simulink model "Follower"  (R2024b)
settings: Solver=ode4  StartTime=0  StopTime=100  FixedStep=0.001  RelTol=1e-3
undefined symbols (not defined in the file or in its folder): DiscIntNeverNeededParam
libraries: simulink x22, vrlib x1
(part 4 of 4)

== matlab function Follower/Ardupilot Attitude Controller/Attitude Controller/input_euler_angle_roll_pitch_euler_rate_yaw()/Feedforward enabled/input shaping/input shaping pitch angle/Square Root Controller1/Square Root Controller ==
  data: err input; correction_rate output; p input; second_ord_lim input; dt input
function correction_rate = sqrt_controller(err, p, second_ord_lim, dt)
% The square root controller
% Code is taken from sqrt_controller(...) in AC_PosControl.cpp.

if (second_ord_lim < 0 || second_ord_lim == 0)
   correction_rate = err * p;
elseif (p == 0)
    % P term is zero, but second order limit is positive
    if (err > 0)
        correction_rate = sqrt(single(2.0) * second_ord_lim * err);
    elseif (err < 0)
        correction_rate = sqrt(single(2.0) * second_ord_lim * -err);
    else
        correction_rate = single(0.0);
    end
else
    % P term and second order limit are positive, hence have been defined
    linear_dist = second_ord_lim / (p * p);
    % Check if error exceeds linear range of controller gain
    if (err > linear_dist)
        correction_rate = sqrt(single(2.0) * second_ord_lim * ( err - (linear_dist / single(2.0)) ));
    elseif (err < -linear_dist)
        correction_rate = -sqrt(single(2.0) * second_ord_lim * ( -err - (linear_dist / single(2.0)) ));
    else
        % Return linearly amplified correction if error is in linear range
        correction_rate = err * p;
    end
end

% Prevent oscillations by over-shooting the error correction in the last
% time step
if (dt ~= 0)
    correction_rate = max( min(correction_rate, abs(err) / dt), -abs(err) / dt);
end

== matlab function Follower/Ardupilot Attitude Controller/Attitude Controller/input_euler_angle_roll_pitch_euler_rate_yaw()/Feedforward enabled/input shaping/input shaping roll angle/Square Root Controller1/Square Root Controller ==
  data: err input; correction_rate output; p input; second_ord_lim input; dt input
function correction_rate = sqrt_controller(err, p, second_ord_lim, dt)
% The square root controller
% Code is taken from sqrt_controller(...) in AC_PosControl.cpp.

if (second_ord_lim < 0 || second_ord_lim == 0)
   correction_rate = err * p;
elseif (p == 0)
    % P term is zero, but second order limit is positive
    if (err > 0)
        correction_rate = sqrt(single(2.0) * second_ord_lim * err);
    elseif (err < 0)
        correction_rate = sqrt(single(2.0) * second_ord_lim * -err);
    else
        correction_rate = single(0.0);
    end
else
    % P term and second order limit are positive, hence have been defined
    linear_dist = second_ord_lim / (p * p);
    % Check if error exceeds linear range of controller gain
    if (err > linear_dist)
        correction_rate = sqrt(single(2.0) * second_ord_lim * ( err - (linear_dist / single(2.0)) ));
    elseif (err < -linear_dist)
        correction_rate = -sqrt(single(2.0) * second_ord_lim * ( -err - (linear_dist / single(2.0)) ));
    else
        % Return linearly amplified correction if error is in linear range
        correction_rate = err * p;
    end
end

% Prevent oscillations by over-shooting the error correction in the last
% time step
if (dt ~= 0)
    correction_rate = max( min(correction_rate, abs(err) / dt), -abs(err) / dt);
end

== matlab function Follower/Ardupilot Attitude Controller/Attitude Controller/input_euler_angle_roll_pitch_euler_rate_yaw()/Feedforward enabled/input shaping/input shaping yaw rate/Square Root Controller/Square Root Controller ==
  data: err input; correction_rate output; p input; second_ord_lim input; dt input
function correction_rate = sqrt_controller(err, p, second_ord_lim, dt)
% The square root controller
% Code is taken from sqrt_controller(...) in AC_PosControl.cpp.

if (second_ord_lim < 0 || second_ord_lim == 0)
   correction_rate = err * p;
elseif (p == 0)
    % P term is zero, but second order limit is positive
    if (err > 0)
        correction_rate = sqrt(single(2.0) * second_ord_lim * err);
    elseif (err < 0)
        correction_rate = sqrt(single(2.0) * second_ord_lim * -err);
    else
        correction_rate = single(0.0);
    end
else
    % P term and second order limit are positive, hence have been defined
    linear_dist = second_ord_lim / (p * p);
    % Check if error exceeds linear range of controller gain
    if (err > linear_dist)
        correction_rate = sqrt(single(2.0) * second_ord_lim * ( err - (linear_dist / single(2.0)) ));
    elseif (err < -linear_dist)
        correction_rate = -sqrt(single(2.0) * second_ord_lim * ( -err - (linear_dist / single(2.0)) ));
    else
        % Return linearly amplified correction if error is in linear range
        correction_rate = err * p;
    end
end

% Prevent oscillations by over-shooting the error correction in the last
% time step
if (dt ~= 0)
    correction_rate = max( min(correction_rate, abs(err) / dt), -abs(err) / dt);
end

== matlab function Follower/Ardupilot Attitude Controller/MATLAB Function4 ==
  data: x input; phi_des output; xdes input; theta_des output; psidot_des output; Ux input; Uy input
function [phi_des, theta_des, psidot_des] = GetDesiredAttitude(x, xdes, Ux, Uy)
% Calculate phi and theta desired based on psi, Ux and Uy and limit them to
% +- pi/3
% xdes = [phi p theta q psi r x xdot y ydot z zdot]
angle_limit = 5*pi/12;

temp1 = Ux * sin(xdes(5)) - Uy * cos(xdes(5));
phi_des = asin(max(min(temp1, sin(angle_limit)), -sin(angle_limit)));

temp2 = (Ux - sin(xdes(1)) * sin(xdes(5))) / (cos(xdes(1)) * cos(xdes(5))); 
theta_des = asin(max(min(temp2, sin(angle_limit)), -sin(angle_limit)));

Kp_psi = 1.0;
psidot_des = Kp_psi * (xdes(5) - x(5));

== matlab function Follower/MATLAB Function5 ==
  data: V output; Z input
function V  = RotorModel(Z)

V = zeros(4,1);
V(1) = Z(1)^2/2;
V(2) = (V(1) + Z(2)^2)/2;
V(3) = Z(3)^2/2;
V(4) = (V(3) + Z(4)^2)/2;

== matlab function Follower/SMC Position Controller/MATLAB Function7 ==
  data: zintg input; x input; Sx output; Sy output; Sz output; Z output; xhat input; xdes input
function [Sx, Sy, Sz, Z] = SlidingSurfaces(zintg, x, xhat, xdes)

% xdes = (phi p theta q psi r x xdot y ydot z zdot)
alpha = 1.5;

z = zeros(12,1);
for i = 1:2:6
    z(i) = x(i) - xdes(i);
    
    % Using ground truth states
    % z(6 + i) = x(6 + i) - xdes(6 + i);
    % Using estimated states
    z(6 + i) = xhat(i) - xdes(6 + i);
end
for j = 2:2:6
    z(j) = x(j) - xdes(j) + alpha*z(j-1);
    
    % Using ground truth states
    % z(6 + j) = x(6 + j) - xdes(6 + j);
    % Using estimated states
    z(6 + j) = xhat(j) - xdes(6 + j);
end
Z = [z(1); z(2); z(3); z(4)];

% Normal SMC
Sx = z(8) + alpha*z(7);
Sy = z(10) + alpha*z(9);
% Sz = z(12) + alpha*z(11);

% Integral SMC
Sz = z(12) + 2*alpha*z(11) + alpha^2 * zintg;

== matlab function Follower/SMC Position Controller/MATLAB Function1 ==
  data: x input; xhat input; xdes input; xdesdot input; U1 output; Ux output; Uy output; Sx input; Sy input; Sz input; k1 output; kx output; ky output
function [U1, Ux, Uy, k1, kx, ky] = PositionController(x, xhat, xdes, xdesdot, Sx, Sy, Sz)

%initializing constants
m = 1.029; g = 9.81;
Cphi = cos(x(1)); Ctheta = cos(x(3));
alpha = 1.5; beta = 1.5; eta = 0.5;

% Thrust Vector Input
% Using ground truth states
% U1 = (m/(Cphi*Ctheta))*(-k1*saturate(Sz, 0.4)+ xdesdot(12) - ...
%                        alpha*(x(12)-xdes(12)) + g);

% Using estimated states
% U1 = (m/(Cphi*Ctheta))*(-k1*saturate(Sz, 0.4)+ xdesdot(12) - ...
%                          alpha*(xhat(6)-xdes(12))  + g);

% Using estimated states + integral control
U1hat = (xdesdot(12) - 2*alpha*(xhat(6)-xdes(12)) ...
                - alpha^2*(xhat(5)-xdes(11)) + g);
k1 = beta * eta + (beta - 1) * abs(U1hat);
U1 = m/(Cphi*Ctheta) * (U1hat - k1 * saturate(Sz, 0.4));

% Apply input saturation
U1 = max(min(U1, 39.0), 0);

%Virtual Input
if U1 == 0
    Ux = 0; Uy = 0;
    kx = 0; ky = 0;
else
    % Using ground truth states
    % Ux = (m/U1)*(-kx*saturate(Sx, 0.75) + xdesdot(8) - alpha*(x(8)-xdes(8)));
    % Uy = (m/U1)*(-ky*saturate(Sy, 0.75) + xdesdot(10) - alpha*(x(10)-xdes(10)));
    
    % Using estimated states
    Uxhat = (xdesdot(8) - alpha*(xhat(2)-xdes(8)));
    Uyhat = (xdesdot(10) - alpha*(xhat(4)-xdes(10)));
    kx = beta * eta + (beta - 1) * abs(Uxhat);
    ky = beta * eta + (beta - 1) * abs(Uyhat);
%     kx = (kx > 2.0) * kx + (kx <= 2.0) * 2.0;
%     ky = (ky > 2.0) * ky + (ky <= 2.0) * 2.0;
    Ux = (m/U1) * (Uxhat - kx * saturate(Sx, 0.5));
    Uy = (m/U1) * (Uyhat - ky * saturate(Sy, 0.5));
end
